simulink model "Pid_controller"  (R2022b)
settings: Solver=FixedStepAuto  StartTime=0.0  StopTime=inf  FixedStep=0.01  RelTol=1e-3
libraries: arduinolib x2, arduinosensorlib x1
settings Model: ExtModeTrigDuration=2  Creator=Sayan  LastModifiedBy=laksh
settings SolverCC: AutoInsertRateTranBlk=on
settings OptimizationCC: EnhancedBackFolding=on  PassReuseOutputArgsAs=Individual arguments  ZeroExternalMemoryAtStartup=off  ZeroInternalMemoryAtStartup=off  MaxStackSize=64  OptimizeBlockOrder=speed  DifferentSizesBufferReuse=on  OptimizationCustomize=off  EfficientTunableParamExpr=on
settings DebuggingCC: ParameterTunabilityLossMsg=error
settings HardwareCC: ProdBitPerInt=16  ProdBitPerPointer=16  ProdBitPerSizeT=16  ProdBitPerPtrDiffT=16  ProdLargestAtomicFloat=None  ProdWordSize=8  ProdHWDeviceType=Atmel->AVR  UseEmbeddedCoderFeatures=off  UseSimulinkCoderFeatures=off
settings SFSimCC: MATLABDynamicMemAlloc=off
settings RTWCC: Description=Embedded Coder  SystemTargetFile=ert.tlc  HardwareBoard=Arduino Uno  TLCOptions=-aInlineSetEventsForThisBaseRateFcn=TLC_FALSE -aSuppressMultiTaskScheduler=TLC_FALSE -aRateBasedStepFcn=1  TemplateMakefile=ert_default_tmf  Toolchain=Arduino AVR  BuildConfiguration=Faster Runs
settings CodeAppCC: ForceParamTrailComments=on  IgnoreCustomStorageClasses=off  OperatorAnnotations=on  SimulinkDataObjDesc=on  SFDataObjDesc=on  MangleLength=10  InsertBlockDesc=on
settings ERTTargetCC: SupportContinuousTime=on  SupportNonInlinedSFcns=on  SupportVariableSizeSignals=on  ExtModeTransport=3  ExtModeStaticAlloc=on  ExtModeAutomaticAllocSize=off  ExtModeStaticAllocSize=250  ExtModeMexFile=ext_xcp  ExtModeIntrfLevel=Level2 - Open

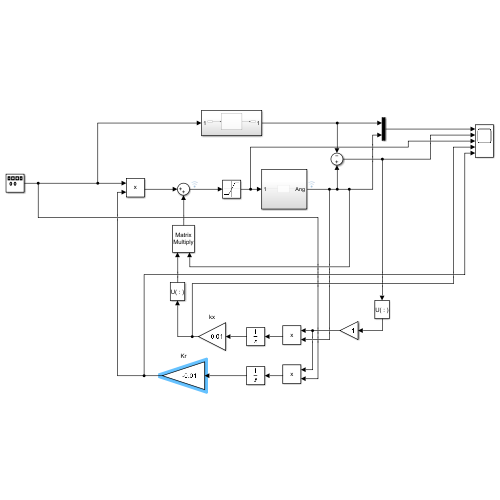
[thumbnail: Simulink's stored preview of the top-level diagram]
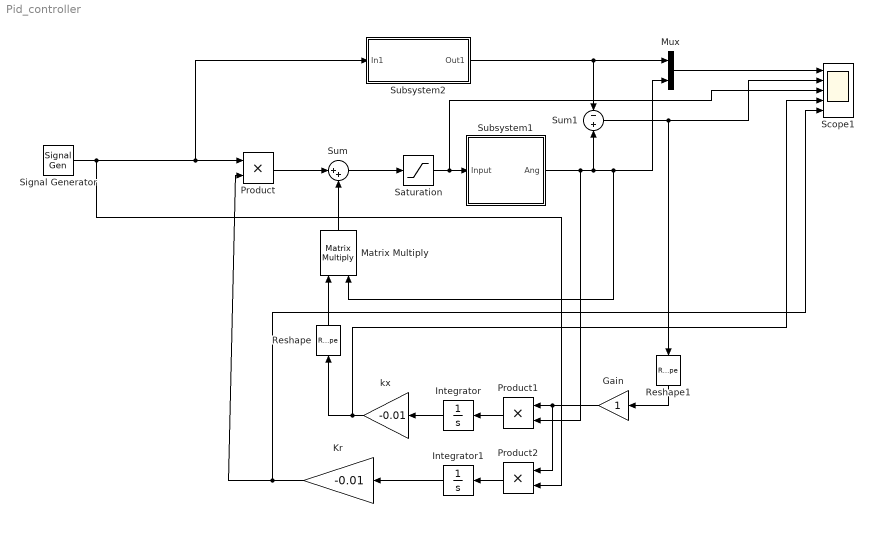
== system Pid_controller ==
  Gain : Gain
  Integrator : Integrator
  Integrator1 : Integrator
  Kr : Gain  Gain=-0.01
  Matrix Multiply : Product  Multiplication=Matrix(*)
  Mux : Mux  Inputs=2
  Product : Product
  Product1 : Product
  Product2 : Product
  Reshape : Reshape
  Reshape1 : Reshape
  Saturation : Saturate  UpperLimit=25  LowerLimit=-25
  Scope1 : Scope  NumInputPorts=5
  Signal Generator : SignalGenerator  WaveForm=square  Amplitude=0  Frequency=0.01
  Subsystem1 : Subsystem
  Subsystem2 : Subsystem
  Sum : Sum  Inputs=|++
  Sum1 : Sum  Inputs=-|+
  kx : Gain  Gain=-0.01
  wires:
  Sum/1 -> Saturation/1
  Integrator1/1 -> Kr/1
  Product1/1 -> Integrator/1
  Mux/1 -> Scope1/1
  Reshape/1 -> Matrix Multiply/1
  Subsystem1/1(Ang) -> Mux/2, Matrix Multiply/2, Sum1/2, Product1/2
  Gain/1 -> Product1/1, Product2/1
  Matrix Multiply/1 -> Sum/2
  Sum1/1 -> Reshape1/1, Scope1/2
  Signal Generator/1 -> Subsystem2/1(In1), Product/1, Product2/2
  Product/1 -> Sum/1
  Reshape1/1 -> Gain/1
  Subsystem2/1(Out1) -> Mux/1, Sum1/1
  Integrator/1 -> kx/1
  Saturation/1 -> Scope1/3, Subsystem1/1(Input)
  kx/1 -> Scope1/4, Reshape/1
  Product2/1 -> Integrator1/1
  Kr/1 -> Scope1/5, Product/2

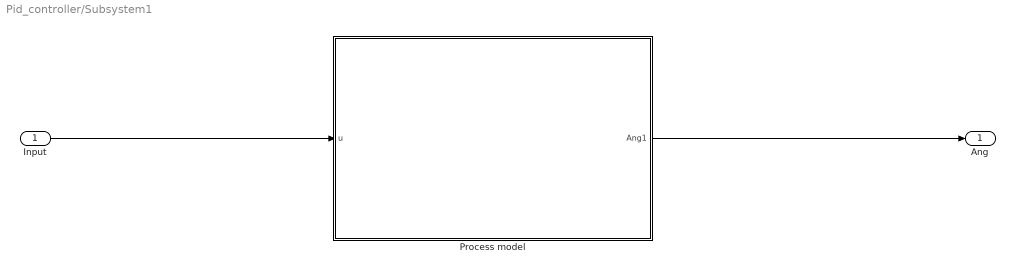
== system Pid_controller/Subsystem1 ==
  Input : Inport
  Process model : Subsystem
  Ang : Outport
  wires:
  Process model/1(Ang1) -> Ang/1
  Input/1 -> Process model/1(u)

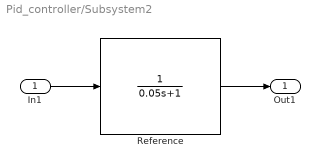
== system Pid_controller/Subsystem2 ==
  In1 : Inport
  Reference : TransferFcn  Denominator=[0.05 1]
  Out1 : Outport
  wires:
  In1/1 -> Reference/1
  Reference/1 -> Out1/1

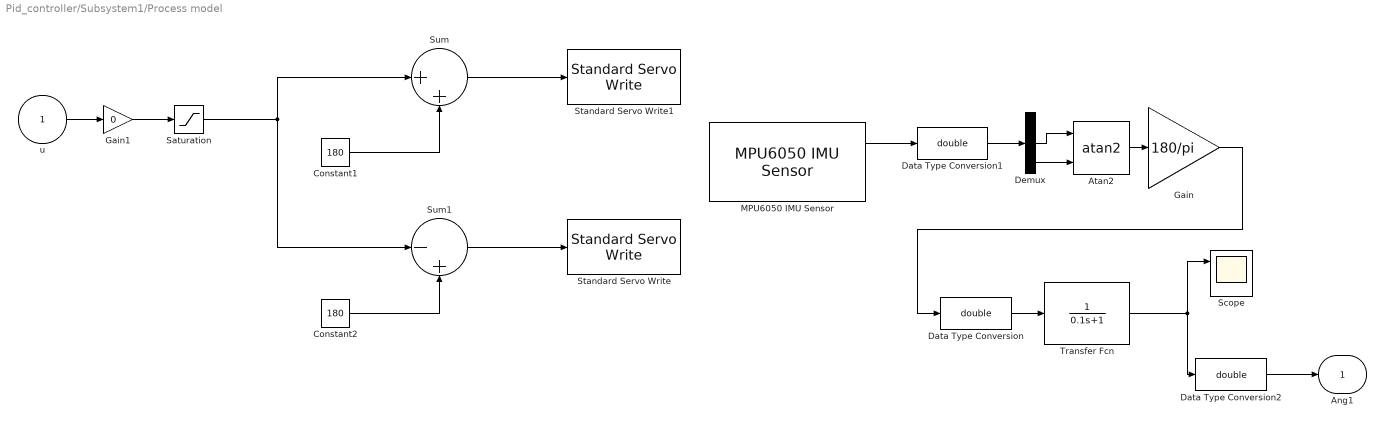
== system Pid_controller/Subsystem1/Process model ==
  u : Inport
  Atan2 : Trigonometry  Operator=atan2
  Constant1 : Constant  Value=180
  Constant2 : Constant  Value=180
  Data Type Conversion : DataTypeConversion  OutDataTypeStr=double  SaturateOnIntegerOverflow=off  RndMeth=Floor
  Data Type Conversion1 : DataTypeConversion  OutDataTypeStr=double  SaturateOnIntegerOverflow=off  RndMeth=Floor
  Data Type Conversion2 : DataTypeConversion  OutDataTypeStr=double  SaturateOnIntegerOverflow=off  RndMeth=Floor
  Demux : Demux  Outputs=3
  Gain : Gain  Gain=180/pi
  Gain1 : Gain  Gain=0
  MPU6050 IMU Sensor : arduinosensorlib/MPU6050 IMU Sensor  SlaveAddress=0x68  Accel=on  AngularRate=on  Temperature=off  Status=off  Timestamp=off  EulerAngles=off  Quat=off  AccelRange=4G  GyroRange=500 dps  DmpOdr=200 Hz  Dlpf=Accelerometer: 184Hz, Gyroscope: 188Hz  spf=1  SampleTime=-1  QueueSizeFactor=1
  Saturation : Saturate  UpperLimit=180  LowerLimit=-180
  Scope : Scope  NumInputPorts=2
  Standard Servo Write : arduinolib/Standard Servo Write  pinNumber=3  ServoIndex=0  blockPlatform=ARDUINO
  Standard Servo Write1 : arduinolib/Standard Servo Write  pinNumber=6  ServoIndex=1  blockPlatform=ARDUINO
  Sum : Sum  Inputs=|++
  Sum1 : Sum  Inputs=|-+
  Transfer Fcn : TransferFcn  Denominator=[0.1 1]
  Ang1 : Outport
  wires:
  MPU6050 IMU Sensor/1 -> Data Type Conversion1/1
  Data Type Conversion1/1 -> Demux/1
  Constant1/1 -> Sum/2
  Sum/1 -> Standard Servo Write1/1
  Sum1/1 -> Standard Servo Write/1
  Demux/2 -> Atan2/1
  Constant2/1 -> Sum1/2
  Demux/3 -> Atan2/2
  Atan2/1 -> Gain/1
  u/1 -> Gain1/1
  Gain/1 -> Data Type Conversion/1
  Transfer Fcn/1 -> Data Type Conversion2/1, Scope/1
  Data Type Conversion/1 -> Transfer Fcn/1
  Saturation/1 -> Sum1/1, Sum/1
  Gain1/1 -> Saturation/1
  Data Type Conversion2/1 -> Ang1/1
